simulink model "engine"  (R2016b)
settings: Solver=VariableStepAuto  StartTime=0.0  StopTime=50  RelTol=1e-3
settings Model: Creator=dell  LastModifiedBy=dell

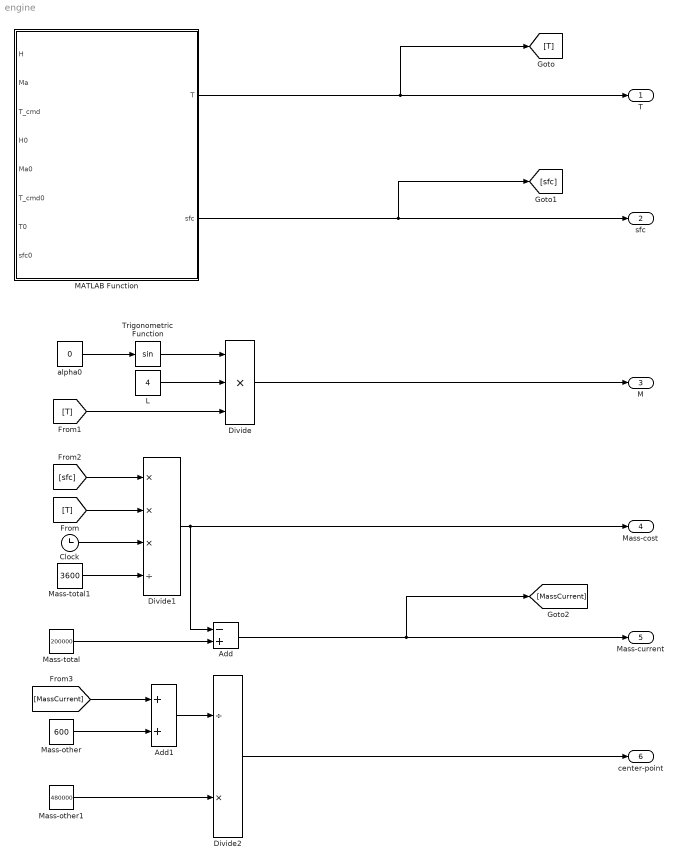
== system engine ==
  Add : Sum  Inputs=-+
  Add1 : Sum
  Clock : Clock
  Divide : Product  Inputs=***
  Divide1 : Product  Inputs=***/
  Divide2 : Product  Inputs=/*
  L : Constant  Value=4
  MATLAB Function : MATLAB Function  TreatAsAtomicUnit=on
  Mass-other : Constant  Value=600
  Mass-other1 : Constant  Value=480000
  Mass-total : Constant  Value=200000
  Mass-total1 : Constant  Value=3600
  Trigonometric Function : Trigonometry
  alpha0 : Constant  Value=0
  T : Outport
  sfc : Outport  Port=2
  M : Outport  Port=3
  Mass-cost : Outport  Port=4
  Mass-current : Outport  Port=5
  center-point : Outport  Port=6
  wires:
  MATLAB Function/1(T) -> T/1, [T]
  alpha0/1 -> Trigonometric Function/1
  Trigonometric Function/1 -> Divide/1
  L/1 -> Divide/2
  Divide/1 -> M/1
  MATLAB Function/2(sfc) -> [sfc], sfc/1
  [T] -> Divide1/2
  Clock/1 -> Divide1/3
  Divide1/1 -> Mass-cost/1, Add/1
  Mass-total/1 -> Add/2
  Add/1 -> [MassCurrent], Mass-current/1
  [T] -> Divide/3
  [sfc] -> Divide1/1
  [MassCurrent] -> Add1/1
  Mass-other/1 -> Add1/2
  Add1/1 -> Divide2/1
  Mass-other1/1 -> Divide2/2
  Divide2/1 -> center-point/1
  Mass-total1/1 -> Divide1/4

== matlab function engine/MATLAB Function ==
  data: H input; T output; Ma input; T_cmd input; H0 input; Ma0 input; T_cmd0 input; T0 input; sfc0 input; sfc output
function [T,sfc] = fcn(H,Ma,T_cmd,H0,Ma0,T_cmd0,T0,sfc0)
[T,sfc]=interpn(Ma0,H0,T_cmd0,T0,sfc0,Ma,H,T_cmd);
end
